simulink model "multiIMU_FES"  (R2021a)
settings: Solver=VariableStepAuto  StartTime=0.0  StopTime=tsim  RelTol=1e-3
undefined symbols (not defined in the file or in its folder): config
libraries: attitude_library x9, sharedtransform x4
settings Model: DataDictionary=bus_definition.sldd  Creator=Laura  LastModifiedBy=Laura

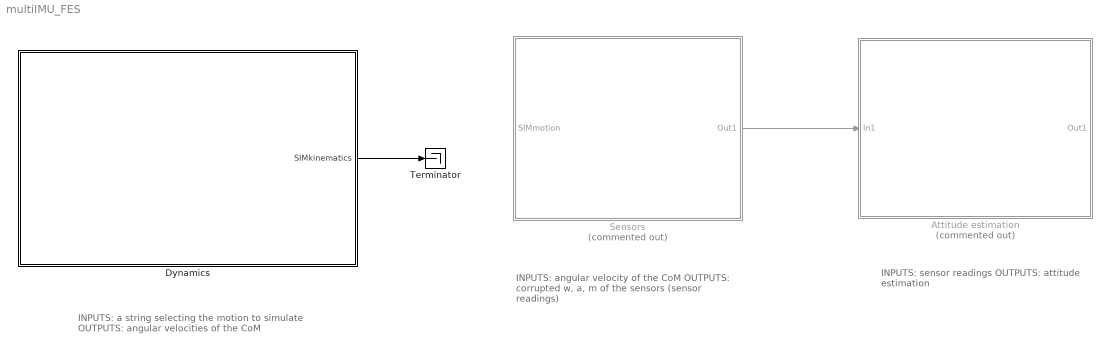
== system multiIMU_FES ==
  note: INPUTS: angular velocity of the CoM
      | OUTPUTS: corrupted w, a, m of the sensors (sensor readings)
  note: INPUTS: a string selecting the motion to simulate
      | OUTPUTS: angular velocities of the CoM
  note: INPUTS: sensor readings
      | OUTPUTS: attitude estimation
  Attitude estimation : Subsystem  Commented=on
  Dynamics : Subsystem
  Sensors : Subsystem  Commented=on
  Terminator : Terminator
  wires:
  Sensors/1(Out1) -> Attitude estimation/1(In1)
  Dynamics/1(SIMkinematics) -> Terminator/1

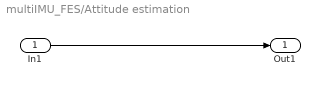
== system multiIMU_FES/Attitude estimation ==
  In1 : Inport
  Out1 : Outport
  wires:
  In1/1 -> Out1/1

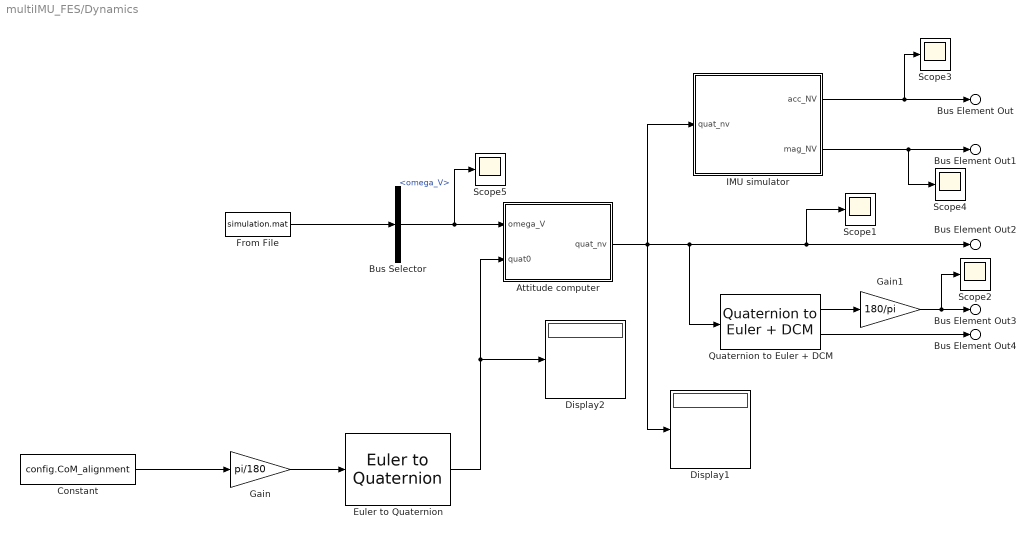
== system multiIMU_FES/Dynamics ==
  Attitude computer : Subsystem
  Bus Selector : BusSelector  OutputSignals=omega_V
  Constant : Constant  Value=config.CoM_alignment  VectorParams1D=off
  Display1 : Display
  Display2 : Display
  Euler to Quaternion : attitude_library/Euler to Quaternion  SystemSampleTime=-1  VariantActivationTime=update diagram  Latency=0  AutoFrameSizeCalculation=off
  From File : FromFile  FileName=simulation.mat  OutDataTypeStr=Bus: SIMin  SampleTime=1/200
  Gain : Gain  Gain=pi/180
  Gain1 : Gain  Gain=180/pi
  IMU simulator : Subsystem
  Quaternion to Euler + DCM : attitude_library/Quaternion to Euler + DCM  SystemSampleTime=-1  VariantActivationTime=update diagram  Latency=0  AutoFrameSizeCalculation=off
  Scope{1..5} (5 alike) : Scope
  Bus Element Out : Outport  PortName=SIMkinematics  Element=acc_V
  Bus Element Out1 : Outport  PortName=SIMkinematics  Element=mag_V
  Bus Element Out2 : Outport  PortName=SIMkinematics  Element=quat_NV
  Bus Element Out4 : Outport  PortName=SIMkinematics  Element=DCM_NV
  Bus Element Out3 : Outport  PortName=SIMkinematics  Element=euler_NV
  wires:
  Gain/1 -> Euler to Quaternion/1
  IMU simulator/1(acc_NV) -> Scope3/1, Bus Element Out/1
  IMU simulator/2(mag_NV) -> Scope4/1, Bus Element Out1/1
  From File/1 -> Bus Selector/1
  Bus Selector/1 -> Scope5/1, Attitude computer/1(omega_V)  "<omega_V>"
  Quaternion to Euler + DCM/1 -> Gain1/1
  Quaternion to Euler + DCM/2 -> Bus Element Out4/1
  Constant/1 -> Gain/1
  Euler to Quaternion/1 -> Display2/1, Attitude computer/2(quat0)
  Attitude computer/1(quat_nv) -> Display1/1, IMU simulator/1(quat_nv), Quaternion to Euler + DCM/1, Scope1/1, Bus Element Out2/1
  Gain1/1 -> Scope2/1, Bus Element Out3/1

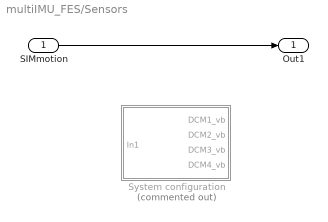
== system multiIMU_FES/Sensors ==
  SIMmotion : Inport
  System configuration : Subsystem  Commented=on
  Out1 : Outport
  wires:
  SIMmotion/1 -> Out1/1

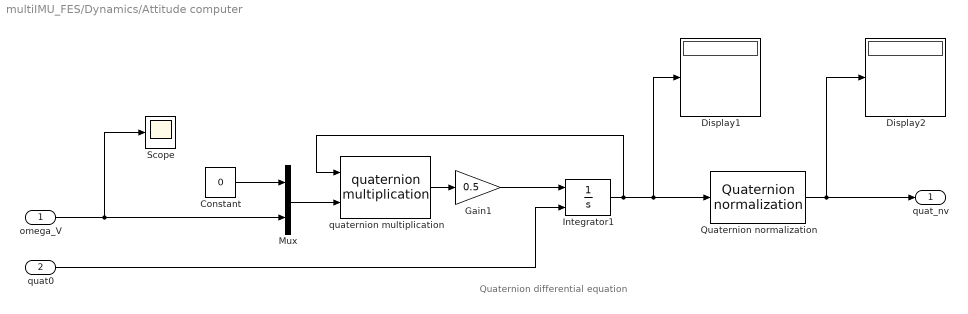
== system multiIMU_FES/Dynamics/Attitude computer ==
  note: Quaternion differential equation
  omega_V : Inport
  quat0 : Inport  Port=2
  Constant : Constant  Value=0
  Display1 : Display
  Display2 : Display
  Gain1 : Gain  Gain=0.5
  Integrator1 : Integrator  InitialConditionSource=external  InitialCondition=[1;0;0;0]
  Mux : Mux  Inputs=2
  Quaternion normalization : attitude_library/Quaternion normalization  SystemSampleTime=-1  VariantActivationTime=update diagram  Latency=0  AutoFrameSizeCalculation=off
  Scope : Scope
  quaternion multiplication : attitude_library/quaternion multiplication  SystemSampleTime=-1  VariantActivationTime=update diagram  Latency=0  AutoFrameSizeCalculation=off
  quat_nv : Outport
  wires:
  Constant/1 -> Mux/1
  Gain1/1 -> Integrator1/1
  omega_V/1 -> Scope/1, Mux/2
  Mux/1 -> quaternion multiplication/2
  Quaternion normalization/1 -> Display2/1, quat_nv/1
  Integrator1/1 -> quaternion multiplication/1, Quaternion normalization/1, Display1/1
  quaternion multiplication/1 -> Gain1/1
  quat0/1 -> Integrator1/2

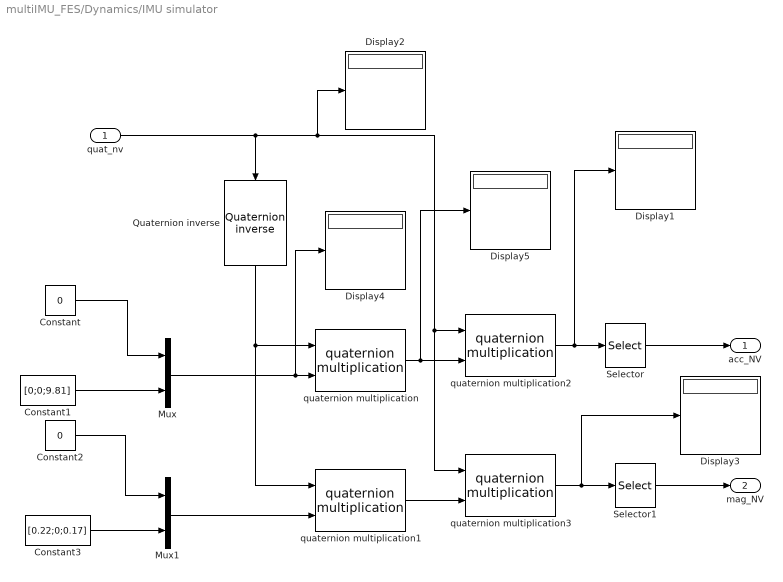
== system multiIMU_FES/Dynamics/IMU simulator ==
  quat_nv : Inport
  Constant : Constant  Value=0
  Constant1 : Constant  Value=[0;0;9.81]
  Constant2 : Constant  Value=0
  Constant3 : Constant  Value=[0.22;0;0.17]
  Display{1..5} (5 alike) : Display
  Mux : Mux  Inputs=2
  Mux1 : Mux  Inputs=2
  Quaternion inverse : attitude_library/Quaternion inverse  SystemSampleTime=-1  VariantActivationTime=update diagram  Latency=0  AutoFrameSizeCalculation=off
      link override Gain: Gain=-1
  Selector : Selector  InputPortWidth=4  IndexOptions=Index vector (dialog)  Indices=[2 3 4]  OutputSizes=1
  Selector1 : Selector  InputPortWidth=4  IndexOptions=Index vector (dialog)  Indices=[2 3 4]  OutputSizes=1
  quaternion multiplication{,1..3} (4 alike) : attitude_library/quaternion multiplication  SystemSampleTime=-1  VariantActivationTime=update diagram  Latency=0  AutoFrameSizeCalculation=off
  acc_NV : Outport
  mag_NV : Outport  Port=2
  wires:
  Constant/1 -> Mux/1
  Constant1/1 -> Mux/2
  quat_nv/1 -> Quaternion inverse/1, Display2/1, quaternion multiplication3/1, quaternion multiplication2/1
  Selector/1 -> acc_NV/1
  Constant2/1 -> Mux1/1
  Selector1/1 -> mag_NV/1
  quaternion multiplication2/1 -> Display1/1, Selector/1
  quaternion multiplication3/1 -> Display3/1, Selector1/1
  quaternion multiplication/1 -> Display5/1, quaternion multiplication2/2
  quaternion multiplication1/1 -> quaternion multiplication3/2
  Quaternion inverse/1 -> quaternion multiplication1/1, quaternion multiplication/1
  Mux1/1 -> quaternion multiplication1/2
  Mux/1 -> quaternion multiplication/2, Display4/1
  Constant3/1 -> Mux1/2

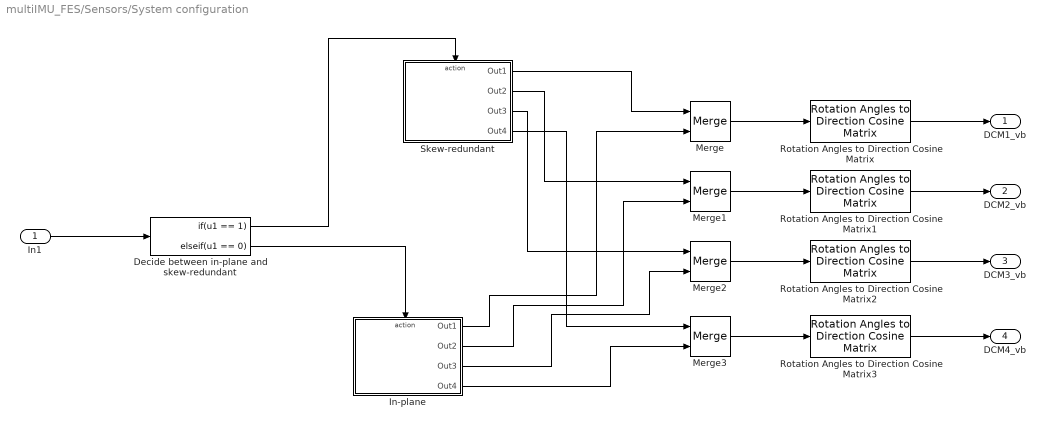
== system multiIMU_FES/Sensors/System configuration ==
  In1 : Inport
  Decide between in-plane and skew-redundant : If  IfExpression=u1 == 1  ElseIfExpressions=u1 == 0  ShowElse=off
  In-plane : Subsystem  TreatAsAtomicUnit=on
  Merge{,1..3} (4 alike) : Merge
  Rotation Angles to Direction Cosine Matrix{,1..3} (4 alike) : sharedtransform/Rotation Angles to Direction Cosine Matrix  rotationOrder=ZYX  aMode=aMode
      settings: SourceProductBaseCode=AE,PW,DR,MT,UV,VE
  Skew-redundant : Subsystem  TreatAsAtomicUnit=on
  DCM1_vb : Outport
  DCM2_vb : Outport  Port=2
  DCM3_vb : Outport  Port=3
  DCM4_vb : Outport  Port=4
  wires:
  Decide between in-plane and skew-redundant/2 -> In-plane/Action
  Skew-redundant/1(Out1) -> Merge/1
  Decide between in-plane and skew-redundant/1 -> Skew-redundant/Action
  In1/1 -> Decide between in-plane and skew-redundant/1
  In-plane/1(Out1) -> Merge/2
  Skew-redundant/2(Out2) -> Merge1/1
  In-plane/2(Out2) -> Merge1/2
  Skew-redundant/3(Out3) -> Merge2/1
  In-plane/3(Out3) -> Merge2/2
  Skew-redundant/4(Out4) -> Merge3/1
  In-plane/4(Out4) -> Merge3/2
  Merge/1 -> Rotation Angles to Direction Cosine Matrix/1
  Merge1/1 -> Rotation Angles to Direction Cosine Matrix1/1
  Merge2/1 -> Rotation Angles to Direction Cosine Matrix2/1
  Merge3/1 -> Rotation Angles to Direction Cosine Matrix3/1
  Rotation Angles to Direction Cosine Matrix/1 -> DCM1_vb/1
  Rotation Angles to Direction Cosine Matrix3/1 -> DCM4_vb/1
  Rotation Angles to Direction Cosine Matrix2/1 -> DCM3_vb/1
  Rotation Angles to Direction Cosine Matrix1/1 -> DCM2_vb/1

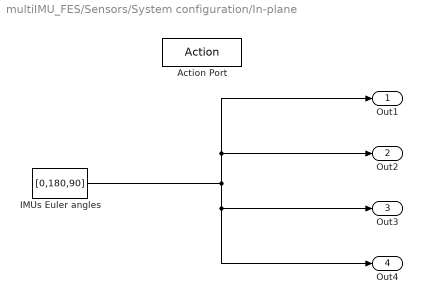
== system multiIMU_FES/Sensors/System configuration/In-plane ==
  Action Port : ActionPort
  IMUs Euler angles : Constant  Value=[0,180,90]
  Out1 : Outport
  Out2 : Outport  Port=2
  Out3 : Outport  Port=3
  Out4 : Outport  Port=4
  wires:
  IMUs Euler angles/1 -> Out3/1, Out4/1, Out2/1, Out1/1

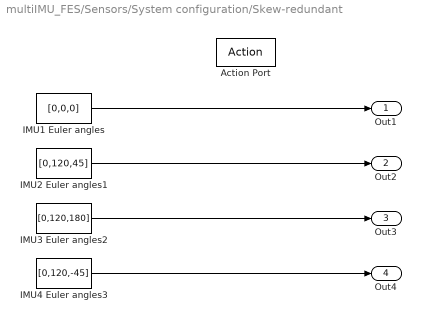
== system multiIMU_FES/Sensors/System configuration/Skew-redundant ==
  Action Port : ActionPort
  IMU1 Euler angles : Constant  Value=[0,0,0]
  IMU2 Euler angles1 : Constant  Value=[0,120,45]
  IMU3 Euler angles2 : Constant  Value=[0,120,180]
  IMU4 Euler angles3 : Constant  Value=[0,120,-45]
  Out1 : Outport
  Out2 : Outport  Port=2
  Out3 : Outport  Port=3
  Out4 : Outport  Port=4
  wires:
  IMU1 Euler angles/1 -> Out1/1
  IMU2 Euler angles1/1 -> Out2/1
  IMU3 Euler angles2/1 -> Out3/1
  IMU4 Euler angles3/1 -> Out4/1
